simulink model "GS_model"  (R2018b)
settings: Solver=ode5  StartTime=0.0  StopTime=SimuStopTime  FixedStep=T_Simu  RelTol=1e-3
InitFcn:
  | Initial
undefined symbols (not defined in the file or in its folder): Aba10, Aba20, aeroCIP2006_S, aeroCIP2006_X, aeroCIP2006_Y, Agl0, Ass_kS, Ass_n1, Ass_n2, Ass_n3, Ass_n4, Ass_Noise, Ass_R, Ass_Resolution, Ass_TmOrder, AssA_Fix_Abs, AssB_Fix_Abs, AssC_Fix_Abs, AssD_Fix_Abs, AssE_Fix_Aps, AssF_Fix_Aps, C, c_max, c_min, Cd, CenterOfFigNX, CenterOfFigNY, CenterOfFigNZ, CenterOfFigP1, CenterOfFigP2, CenterOfFigPX, CenterOfFigPY, CenterOfFigPZ, Cmu, Crou, DEG2RAD, DiscIntNeverNeededParam, Eg_Dir, Eg_F, Eg_PrepareTime, Eg_r_L_L, Fw_Abf, Fw_Hmax, Fw_J, Fw_Spd0, Fw_Tmax, git_hash_BaseLine, git_hash_Project, Gnss_Noise_Pos, Gnss_Noise_Vel, Gnss_PropgationTime, GyroA_Fix_Abg, GyroA_Noise, GyroB_Fix_Abg, GyroB_Noise, GyroC_Fix_Abg, GyroC_Noise, GyroD_Fix_Abg, GyroD_Noise, h ... (+94)
libraries: simulink x308, sharedutil x46, aerolibutil x37, sharedtransform x31, vrlib x14, aerolibgravity2 x2
(part 6 of 20)

== system GS_model/Subsystem2/Subsystem/Actuator/Engine/Subsystem1/Subsystem ==
  note: Dir_Choice/Switch/X/Y/Z
  Eg_Dir0 : Inport
  Eg_Dir_Set : Inport  Port=2
  Num : Inport  Port=3
  Compare To Constant : simulink/Logic and Bit Operations/Compare To Constant  relop===  const=0  OutDataTypeStr=boolean
  Demux : Demux  Outputs=[1;4]
  Demux5 : Demux  Outputs=[1;3]
  Logical Operator : Logic  Operator=OR  AllPortsSameDT=off  OutDataTypeStr=boolean
  Normalize Vector : vrlib/Utilities/Normalize Vector  maxzero=0
  Relational Operator1 : RelationalOperator  Operator===  OutDataTypeStr=boolean  RndMeth=Simplest
  Switch : Switch  Criteria=u2 > Threshold
  Triggered Subsystem1 : Subsystem  TreatAsAtomicUnit=on
      mask Display: disp('FWChoice')
  Eg_Dir : Outport
  wires:
  Normalize Vector/1 -> Eg_Dir/1
  Relational Operator1/1 -> Logical Operator/1
  Compare To Constant/1 -> Logical Operator/2
  Eg_Dir_Set/1 -> Demux/1
  Demux5/1 -> Switch/2
  Eg_Dir0/1 -> Switch/3
  Demux/2 -> Triggered Subsystem1/1(In1)
  Switch/1 -> Normalize Vector/1
  Logical Operator/1 -> Triggered Subsystem1/Enable
  Triggered Subsystem1/1(Out1) -> Demux5/1
  Num/1 -> Relational Operator1/1
  Demux5/2 -> Switch/1
  Demux/1 -> Compare To Constant/1, Relational Operator1/2

== system GS_model/Subsystem2/Subsystem/Actuator/Engine/Subsystem1/Subsystem1 ==
  note: F_Choice/Switch/Value
  Eg_F0 : Inport
  Eg_F_Set : Inport  Port=2
  Num : Inport  Port=3
  Compare To Constant : simulink/Logic and Bit Operations/Compare To Constant  relop===  const=0  OutDataTypeStr=boolean
  Demux : Demux  Outputs=[1;2]
  Demux5 : Demux  Outputs=[1;1]
  Logical Operator : Logic  Operator=OR  AllPortsSameDT=off  OutDataTypeStr=boolean
  Relational Operator1 : RelationalOperator  Operator===  OutDataTypeStr=boolean  RndMeth=Simplest
  Switch : Switch  Criteria=u2 > Threshold
  Triggered Subsystem1 : Subsystem  TreatAsAtomicUnit=on
      mask Display: disp('FWChoice')
  Eg_F : Outport
  wires:
  Demux/1 -> Relational Operator1/2, Compare To Constant/1
  Demux5/2 -> Switch/1
  Num/1 -> Relational Operator1/1
  Triggered Subsystem1/1(Out1) -> Demux5/1
  Logical Operator/1 -> Triggered Subsystem1/Enable
  Switch/1 -> Eg_F/1
  Demux/2 -> Triggered Subsystem1/1(In1)
  Eg_F0/1 -> Switch/3
  Demux5/1 -> Switch/2
  Eg_F_Set/1 -> Demux/1
  Compare To Constant/1 -> Logical Operator/2
  Relational Operator1/1 -> Logical Operator/1

== system GS_model/Subsystem2/Subsystem/Actuator/Engine/Subsystem1/Subsystem2 ==
  note: FirePause_Choice/Switch/Value
  Eg_F_Set : Inport
  Num : Inport  Port=2
  Compare To Constant : simulink/Logic and Bit Operations/Compare To Constant  relop===  const=0  OutDataTypeStr=boolean
  Demux : Demux  Outputs=[1;2]
  Logical Operator : Logic  Operator=OR  AllPortsSameDT=off  OutDataTypeStr=boolean
  Relational Operator1 : RelationalOperator  Operator===  OutDataTypeStr=boolean  RndMeth=Simplest
  Triggered Subsystem1 : Subsystem  TreatAsAtomicUnit=on
      mask Display: disp('FWChoice')
  Eg_FirePause : Outport
  wires:
  Relational Operator1/1 -> Logical Operator/1
  Compare To Constant/1 -> Logical Operator/2
  Eg_F_Set/1 -> Demux/1
  Demux/2 -> Triggered Subsystem1/1(In1)
  Logical Operator/1 -> Triggered Subsystem1/Enable
  Triggered Subsystem1/1(Out1) -> Eg_FirePause/1
  Num/1 -> Relational Operator1/1
  Demux/1 -> Compare To Constant/1, Relational Operator1/2

== system GS_model/Subsystem2/Subsystem/Actuator/FlyWheel/FwAModel1/FWDataSourceChoice ==
  note: 1 -- FW_Spd_422
      | 2 -- FW_Spd_UDP
      | 3 -- FW_Spd_FC
      |
      | 4 -- FW_T_422
      | 5 -- FW_T_UDP
      | 6 -- FW_T_FC
      |
      | 7 -- FW_Mode_422
      | 8 -- FW_Mode_UDP
      | 9 -- FW_Mode_FC
  FW_Cmd : Inport
  TC_FW_DelaySet : Inport  Port=2
  DelayModel : Subsystem
  Demux : Demux  Outputs=3
  Mux1 : Mux  Inputs=3
  Cmd_Mode/Spd/T : Outport
  Cmd_Mode : Outport  Port=2
  wires:
  Mux1/1 -> Cmd_Mode/Spd/T/1
  DelayModel/3(Cmd_T) -> Mux1/3
  DelayModel/1(Cmd_Mode) -> Mux1/1, Cmd_Mode/1
  DelayModel/2(Cmd_Spd) -> Mux1/2
  TC_FW_DelaySet/1 -> DelayModel/1(TC_FW_Delay)
  FW_Cmd/1 -> Demux/1
  Demux/3 -> DelayModel/4(FW_Cmd_T)
  Demux/2 -> DelayModel/3(FW_Cmd_Spd)
  Demux/1 -> DelayModel/2(FW_Cmd_Mode)

== system GS_model/Subsystem2/Subsystem/Actuator/FlyWheel/FwAModel1/FWMath&ErrModel ==
  Cmd_Mode : Inport
  TC_FW_TSet : Inport  Port=2
  TC_FW_SpdSet : Inport  Port=3
  TC_FW_ModeSet : Inport  Port=4
  TC_FWErr_Spd_Op : Inport  Port=5
  TC_FWErr_T_Op : Inport  Port=6
  FwSpd : Inport  Port=7
  FwT : Inport  Port=8
  FWNum : Inport  Port=9
  Mux : Mux  Inputs=3
  Subsystem1 : Subsystem
      mask Display: disp('FWTErrModel')
  Subsystem2 : Subsystem
      mask Display: disp('FWSpdErrModel')
  Subsystem4 : Subsystem
      mask Display: disp('FWModeErrModel')
  TM_FW : Outport
  Dyn_FW_T : Outport  Port=2
  Dyn_FW_Spd : Outport  Port=3
  wires:
  FwSpd/1 -> Subsystem2/1(Fb_FW_Spd), Dyn_FW_Spd/1
  TC_FW_TSet/1 -> Subsystem1/2(TC_FW_TSet)
  TC_FW_SpdSet/1 -> Subsystem2/2(TC_FW_SpdSet)
  TC_FW_ModeSet/1 -> Subsystem4/3(TC_FW_ModeSet)
  FwT/1 -> Subsystem1/1(Fb_FW_T), Dyn_FW_T/1
  Cmd_Mode/1 -> Subsystem4/2(FW_Mode)
  TC_FWErr_Spd_Op/1 -> Subsystem2/4(TC_FWErr_SpdOp)
  TC_FWErr_T_Op/1 -> Subsystem1/4(TC_FWErr_TOp)
  Mux/1 -> TM_FW/1
  Subsystem2/1(TM_FW_Spd) -> Mux/2
  Subsystem4/1(Fb_FW_Mode) -> Mux/1
  Subsystem1/1(TM_FW_T) -> Mux/3
  FWNum/1 -> Subsystem1/3(FWNum), Subsystem2/3(FWNum), Subsystem4/1(FWNum)

== system GS_model/Subsystem2/Subsystem/Actuator/FlyWheel/FwAModel2/FWDataSourceChoice ==
  note: 1 -- FW_Spd_422
      | 2 -- FW_Spd_UDP
      | 3 -- FW_Spd_FC
      |
      | 4 -- FW_T_422
      | 5 -- FW_T_UDP
      | 6 -- FW_T_FC
      |
      | 7 -- FW_Mode_422
      | 8 -- FW_Mode_UDP
      | 9 -- FW_Mode_FC
  FW_Cmd : Inport
  TC_FW_DelaySet : Inport  Port=2
  DelayModel : Subsystem
  Demux : Demux  Outputs=3
  Mux1 : Mux  Inputs=3
  Cmd_Mode/Spd/T : Outport
  Cmd_Mode : Outport  Port=2
  wires:
  Demux/1 -> DelayModel/2(FW_Cmd_Mode)
  Demux/2 -> DelayModel/3(FW_Cmd_Spd)
  Demux/3 -> DelayModel/4(FW_Cmd_T)
  FW_Cmd/1 -> Demux/1
  TC_FW_DelaySet/1 -> DelayModel/1(TC_FW_Delay)
  DelayModel/2(Cmd_Spd) -> Mux1/2
  DelayModel/1(Cmd_Mode) -> Cmd_Mode/1, Mux1/1
  DelayModel/3(Cmd_T) -> Mux1/3
  Mux1/1 -> Cmd_Mode/Spd/T/1

== system GS_model/Subsystem2/Subsystem/Actuator/FlyWheel/FwAModel2/FWMath&ErrModel ==
  Cmd_Mode : Inport
  TC_FW_TSet : Inport  Port=2
  TC_FW_SpdSet : Inport  Port=3
  TC_FW_ModeSet : Inport  Port=4
  TC_FWErr_Spd_Op : Inport  Port=5
  TC_FWErr_T_Op : Inport  Port=6
  FwSpd : Inport  Port=7
  FwT : Inport  Port=8
  FWNum : Inport  Port=9
  Mux : Mux  Inputs=3
  Subsystem1 : Subsystem
      mask Display: disp('FWTErrModel')
  Subsystem2 : Subsystem
      mask Display: disp('FWSpdErrModel')
  Subsystem4 : Subsystem
      mask Display: disp('FWModeErrModel')
  TM_FW : Outport
  Dyn_FW_T : Outport  Port=2
  Dyn_FW_Spd : Outport  Port=3
  wires:
  FWNum/1 -> Subsystem4/1(FWNum), Subsystem2/3(FWNum), Subsystem1/3(FWNum)
  Subsystem1/1(TM_FW_T) -> Mux/3
  Subsystem4/1(Fb_FW_Mode) -> Mux/1
  Subsystem2/1(TM_FW_Spd) -> Mux/2
  Mux/1 -> TM_FW/1
  TC_FWErr_T_Op/1 -> Subsystem1/4(TC_FWErr_TOp)
  TC_FWErr_Spd_Op/1 -> Subsystem2/4(TC_FWErr_SpdOp)
  Cmd_Mode/1 -> Subsystem4/2(FW_Mode)
  FwT/1 -> Dyn_FW_T/1, Subsystem1/1(Fb_FW_T)
  TC_FW_ModeSet/1 -> Subsystem4/3(TC_FW_ModeSet)
  TC_FW_SpdSet/1 -> Subsystem2/2(TC_FW_SpdSet)
  TC_FW_TSet/1 -> Subsystem1/2(TC_FW_TSet)
  FwSpd/1 -> Dyn_FW_Spd/1, Subsystem2/1(Fb_FW_Spd)

== system GS_model/Subsystem2/Subsystem/Actuator/FlyWheel/FwAModel3/FWDataSourceChoice ==
  note: 1 -- FW_Spd_422
      | 2 -- FW_Spd_UDP
      | 3 -- FW_Spd_FC
      |
      | 4 -- FW_T_422
      | 5 -- FW_T_UDP
      | 6 -- FW_T_FC
      |
      | 7 -- FW_Mode_422
      | 8 -- FW_Mode_UDP
      | 9 -- FW_Mode_FC
  FW_Cmd : Inport
  TC_FW_DelaySet : Inport  Port=2
  DelayModel : Subsystem
  Demux : Demux  Outputs=3
  Mux1 : Mux  Inputs=3
  Cmd_Mode/Spd/T : Outport
  Cmd_Mode : Outport  Port=2
  wires:
  Mux1/1 -> Cmd_Mode/Spd/T/1
  DelayModel/3(Cmd_T) -> Mux1/3
  DelayModel/1(Cmd_Mode) -> Mux1/1, Cmd_Mode/1
  DelayModel/2(Cmd_Spd) -> Mux1/2
  TC_FW_DelaySet/1 -> DelayModel/1(TC_FW_Delay)
  FW_Cmd/1 -> Demux/1
  Demux/3 -> DelayModel/4(FW_Cmd_T)
  Demux/2 -> DelayModel/3(FW_Cmd_Spd)
  Demux/1 -> DelayModel/2(FW_Cmd_Mode)

== system GS_model/Subsystem2/Subsystem/Actuator/FlyWheel/FwAModel3/FWMath&ErrModel ==
  Cmd_Mode : Inport
  TC_FW_TSet : Inport  Port=2
  TC_FW_SpdSet : Inport  Port=3
  TC_FW_ModeSet : Inport  Port=4
  TC_FWErr_Spd_Op : Inport  Port=5
  TC_FWErr_T_Op : Inport  Port=6
  FwSpd : Inport  Port=7
  FwT : Inport  Port=8
  FWNum : Inport  Port=9
  Mux : Mux  Inputs=3
  Subsystem1 : Subsystem
      mask Display: disp('FWTErrModel')
  Subsystem2 : Subsystem
      mask Display: disp('FWSpdErrModel')
  Subsystem4 : Subsystem
      mask Display: disp('FWModeErrModel')
  TM_FW : Outport
  Dyn_FW_T : Outport  Port=2
  Dyn_FW_Spd : Outport  Port=3
  wires:
  FwSpd/1 -> Subsystem2/1(Fb_FW_Spd), Dyn_FW_Spd/1
  TC_FW_TSet/1 -> Subsystem1/2(TC_FW_TSet)
  TC_FW_SpdSet/1 -> Subsystem2/2(TC_FW_SpdSet)
  TC_FW_ModeSet/1 -> Subsystem4/3(TC_FW_ModeSet)
  FwT/1 -> Subsystem1/1(Fb_FW_T), Dyn_FW_T/1
  Cmd_Mode/1 -> Subsystem4/2(FW_Mode)
  TC_FWErr_Spd_Op/1 -> Subsystem2/4(TC_FWErr_SpdOp)
  TC_FWErr_T_Op/1 -> Subsystem1/4(TC_FWErr_TOp)
  Mux/1 -> TM_FW/1
  Subsystem2/1(TM_FW_Spd) -> Mux/2
  Subsystem4/1(Fb_FW_Mode) -> Mux/1
  Subsystem1/1(TM_FW_T) -> Mux/3
  FWNum/1 -> Subsystem1/3(FWNum), Subsystem2/3(FWNum), Subsystem4/1(FWNum)

== system GS_model/Subsystem2/Subsystem/Actuator/FlyWheel/FwAModel4/FWDataSourceChoice ==
  note: 1 -- FW_Spd_422
      | 2 -- FW_Spd_UDP
      | 3 -- FW_Spd_FC
      |
      | 4 -- FW_T_422
      | 5 -- FW_T_UDP
      | 6 -- FW_T_FC
      |
      | 7 -- FW_Mode_422
      | 8 -- FW_Mode_UDP
      | 9 -- FW_Mode_FC
  FW_Cmd : Inport
  TC_FW_DelaySet : Inport  Port=2
  DelayModel : Subsystem
  Demux : Demux  Outputs=3
  Mux1 : Mux  Inputs=3
  Cmd_Mode/Spd/T : Outport
  Cmd_Mode : Outport  Port=2
  wires:
  Demux/1 -> DelayModel/2(FW_Cmd_Mode)
  Demux/2 -> DelayModel/3(FW_Cmd_Spd)
  Demux/3 -> DelayModel/4(FW_Cmd_T)
  FW_Cmd/1 -> Demux/1
  TC_FW_DelaySet/1 -> DelayModel/1(TC_FW_Delay)
  DelayModel/2(Cmd_Spd) -> Mux1/2
  DelayModel/1(Cmd_Mode) -> Cmd_Mode/1, Mux1/1
  DelayModel/3(Cmd_T) -> Mux1/3
  Mux1/1 -> Cmd_Mode/Spd/T/1

== system GS_model/Subsystem2/Subsystem/Actuator/FlyWheel/FwAModel4/FWMath&ErrModel ==
  Cmd_Mode : Inport
  TC_FW_TSet : Inport  Port=2
  TC_FW_SpdSet : Inport  Port=3
  TC_FW_ModeSet : Inport  Port=4
  TC_FWErr_Spd_Op : Inport  Port=5
  TC_FWErr_T_Op : Inport  Port=6
  FwSpd : Inport  Port=7
  FwT : Inport  Port=8
  FWNum : Inport  Port=9
  Mux : Mux  Inputs=3
  Subsystem1 : Subsystem
      mask Display: disp('FWTErrModel')
  Subsystem2 : Subsystem
      mask Display: disp('FWSpdErrModel')
  Subsystem4 : Subsystem
      mask Display: disp('FWModeErrModel')
  TM_FW : Outport
  Dyn_FW_T : Outport  Port=2
  Dyn_FW_Spd : Outport  Port=3
  wires:
  FWNum/1 -> Subsystem4/1(FWNum), Subsystem2/3(FWNum), Subsystem1/3(FWNum)
  Subsystem1/1(TM_FW_T) -> Mux/3
  Subsystem4/1(Fb_FW_Mode) -> Mux/1
  Subsystem2/1(TM_FW_Spd) -> Mux/2
  Mux/1 -> TM_FW/1
  TC_FWErr_T_Op/1 -> Subsystem1/4(TC_FWErr_TOp)
  TC_FWErr_Spd_Op/1 -> Subsystem2/4(TC_FWErr_SpdOp)
  Cmd_Mode/1 -> Subsystem4/2(FW_Mode)
  FwT/1 -> Dyn_FW_T/1, Subsystem1/1(Fb_FW_T)
  TC_FW_ModeSet/1 -> Subsystem4/3(TC_FW_ModeSet)
  TC_FW_SpdSet/1 -> Subsystem2/2(TC_FW_SpdSet)
  TC_FW_TSet/1 -> Subsystem1/2(TC_FW_TSet)
  FwSpd/1 -> Dyn_FW_Spd/1, Subsystem2/1(Fb_FW_Spd)

== system GS_model/Subsystem2/Subsystem/Actuator/FlyWheel/FwAModel5/FWDataSourceChoice ==
  note: 1 -- FW_Spd_422
      | 2 -- FW_Spd_UDP
      | 3 -- FW_Spd_FC
      |
      | 4 -- FW_T_422
      | 5 -- FW_T_UDP
      | 6 -- FW_T_FC
      |
      | 7 -- FW_Mode_422
      | 8 -- FW_Mode_UDP
      | 9 -- FW_Mode_FC
  FW_Cmd : Inport
  TC_FW_DelaySet : Inport  Port=2
  DelayModel : Subsystem
  Demux : Demux  Outputs=3
  Mux1 : Mux  Inputs=3
  Cmd_Mode/Spd/T : Outport
  Cmd_Mode : Outport  Port=2
  wires:
  Mux1/1 -> Cmd_Mode/Spd/T/1
  DelayModel/3(Cmd_T) -> Mux1/3
  DelayModel/1(Cmd_Mode) -> Mux1/1, Cmd_Mode/1
  DelayModel/2(Cmd_Spd) -> Mux1/2
  TC_FW_DelaySet/1 -> DelayModel/1(TC_FW_Delay)
  FW_Cmd/1 -> Demux/1
  Demux/3 -> DelayModel/4(FW_Cmd_T)
  Demux/2 -> DelayModel/3(FW_Cmd_Spd)
  Demux/1 -> DelayModel/2(FW_Cmd_Mode)

== system GS_model/Subsystem2/Subsystem/Actuator/FlyWheel/FwAModel5/FWMath&ErrModel ==
  Cmd_Mode : Inport
  TC_FW_TSet : Inport  Port=2
  TC_FW_SpdSet : Inport  Port=3
  TC_FW_ModeSet : Inport  Port=4
  TC_FWErr_Spd_Op : Inport  Port=5
  TC_FWErr_T_Op : Inport  Port=6
  FwSpd : Inport  Port=7
  FwT : Inport  Port=8
  FWNum : Inport  Port=9
  Mux : Mux  Inputs=3
  Subsystem1 : Subsystem
      mask Display: disp('FWTErrModel')
  Subsystem2 : Subsystem
      mask Display: disp('FWSpdErrModel')
  Subsystem4 : Subsystem
      mask Display: disp('FWModeErrModel')
  TM_FW : Outport
  Dyn_FW_T : Outport  Port=2
  Dyn_FW_Spd : Outport  Port=3
  wires:
  FwSpd/1 -> Subsystem2/1(Fb_FW_Spd), Dyn_FW_Spd/1
  TC_FW_TSet/1 -> Subsystem1/2(TC_FW_TSet)
  TC_FW_SpdSet/1 -> Subsystem2/2(TC_FW_SpdSet)
  TC_FW_ModeSet/1 -> Subsystem4/3(TC_FW_ModeSet)
  FwT/1 -> Subsystem1/1(Fb_FW_T), Dyn_FW_T/1
  Cmd_Mode/1 -> Subsystem4/2(FW_Mode)
  TC_FWErr_Spd_Op/1 -> Subsystem2/4(TC_FWErr_SpdOp)
  TC_FWErr_T_Op/1 -> Subsystem1/4(TC_FWErr_TOp)
  Mux/1 -> TM_FW/1
  Subsystem2/1(TM_FW_Spd) -> Mux/2
  Subsystem4/1(Fb_FW_Mode) -> Mux/1
  Subsystem1/1(TM_FW_T) -> Mux/3
  FWNum/1 -> Subsystem1/3(FWNum), Subsystem2/3(FWNum), Subsystem4/1(FWNum)

== system GS_model/Subsystem2/Subsystem/Actuator/FlyWheel/FwAModel6/FWDataSourceChoice ==
  note: 1 -- FW_Spd_422
      | 2 -- FW_Spd_UDP
      | 3 -- FW_Spd_FC
      |
      | 4 -- FW_T_422
      | 5 -- FW_T_UDP
      | 6 -- FW_T_FC
      |
      | 7 -- FW_Mode_422
      | 8 -- FW_Mode_UDP
      | 9 -- FW_Mode_FC
  FW_Cmd : Inport
  TC_FW_DelaySet : Inport  Port=2
  DelayModel : Subsystem
  Demux : Demux  Outputs=3
  Mux1 : Mux  Inputs=3
  Cmd_Mode/Spd/T : Outport
  Cmd_Mode : Outport  Port=2
  wires:
  Demux/1 -> DelayModel/2(FW_Cmd_Mode)
  Demux/2 -> DelayModel/3(FW_Cmd_Spd)
  Demux/3 -> DelayModel/4(FW_Cmd_T)
  FW_Cmd/1 -> Demux/1
  TC_FW_DelaySet/1 -> DelayModel/1(TC_FW_Delay)
  DelayModel/2(Cmd_Spd) -> Mux1/2
  DelayModel/1(Cmd_Mode) -> Cmd_Mode/1, Mux1/1
  DelayModel/3(Cmd_T) -> Mux1/3
  Mux1/1 -> Cmd_Mode/Spd/T/1

== system GS_model/Subsystem2/Subsystem/Actuator/FlyWheel/FwAModel6/FWMath&ErrModel ==
  Cmd_Mode : Inport
  TC_FW_TSet : Inport  Port=2
  TC_FW_SpdSet : Inport  Port=3
  TC_FW_ModeSet : Inport  Port=4
  TC_FWErr_Spd_Op : Inport  Port=5
  TC_FWErr_T_Op : Inport  Port=6
  FwSpd : Inport  Port=7
  FwT : Inport  Port=8
  FWNum : Inport  Port=9
  Mux : Mux  Inputs=3
  Subsystem1 : Subsystem
      mask Display: disp('FWTErrModel')
  Subsystem2 : Subsystem
      mask Display: disp('FWSpdErrModel')
  Subsystem4 : Subsystem
      mask Display: disp('FWModeErrModel')
  TM_FW : Outport
  Dyn_FW_T : Outport  Port=2
  Dyn_FW_Spd : Outport  Port=3
  wires:
  FWNum/1 -> Subsystem4/1(FWNum), Subsystem2/3(FWNum), Subsystem1/3(FWNum)
  Subsystem1/1(TM_FW_T) -> Mux/3
  Subsystem4/1(Fb_FW_Mode) -> Mux/1
  Subsystem2/1(TM_FW_Spd) -> Mux/2
  Mux/1 -> TM_FW/1
  TC_FWErr_T_Op/1 -> Subsystem1/4(TC_FWErr_TOp)
  TC_FWErr_Spd_Op/1 -> Subsystem2/4(TC_FWErr_SpdOp)
  Cmd_Mode/1 -> Subsystem4/2(FW_Mode)
  FwT/1 -> Dyn_FW_T/1, Subsystem1/1(Fb_FW_T)
  TC_FW_ModeSet/1 -> Subsystem4/3(TC_FW_ModeSet)
  TC_FW_SpdSet/1 -> Subsystem2/2(TC_FW_SpdSet)
  TC_FW_TSet/1 -> Subsystem1/2(TC_FW_TSet)
  FwSpd/1 -> Dyn_FW_Spd/1, Subsystem2/1(Fb_FW_Spd)

== system GS_model/Subsystem2/Subsystem/Actuator/FlyWheel/FwAModel7/FwMathModel ==
  note: 1--转矩模式
      | 2--转速模式
  Cmd_Mode : Inport
  Cmd_Spd : Inport  Port=2
  Cmd_T : Inport  Port=3
  Reset : Inport  Port=4
  FwH0 : Inport  Port=5
  Tc_Fw_FricCoff : Inport  Port=6
  10mN--6000rpm : Gain  Gain=0.01./Fw_Hmax
  Compare To Constant : simulink/Logic and Bit Operations/Compare To Constant  relop===  const=2.0  OutDataTypeStr=boolean
  Compare To Constant1 : simulink/Logic and Bit Operations/Compare To Constant  relop===  const=1.0  OutDataTypeStr=boolean
  Data Type Conversion : DataTypeConversion  OutDataTypeStr=double
  Data Type Conversion1 : DataTypeConversion  OutDataTypeStr=double
  Gain2 : Gain  Gain=1./Fw_J
  Gain3 : Gain  Gain=1./Fw_J
  Integrator Limited1 : Integrator  ExternalReset=level  InitialConditionSource=external  LimitOutput=on  UpperSaturationLimit=Fw_Hmax  LowerSaturationLimit=-Fw_Hmax
  K : Gain  Gain=Fw_J  SaturateOnIntegerOverflow=on  OutDataTypeStr=Inherit: Same as input  ParamDataTypeStr=Inherit: Same as input
  Memory : Memory  InheritSampleTime=on
  Product : Product
  Product1 : Product
  Product2 : Product
  RPM2RadPerSec : Gain  Gain=RPM2RadPerSec  SaturateOnIntegerOverflow=on  OutDataTypeStr=Inherit: Same as input  ParamDataTypeStr=Inherit: Same as input
  RadPerSec2RPM : Gain  Gain=RadPerSec2RPM  SaturateOnIntegerOverflow=on  OutDataTypeStr=Inherit: Same as input  ParamDataTypeStr=Inherit: Same as input
  Sum : Sum  Inputs=|+-  SaturateOnIntegerOverflow=on
  Sum1 : Sum  Inputs=++|
  Sum2 : Sum  Inputs=|+-  SaturateOnIntegerOverflow=on
  Sum3 : Sum  Inputs=|+-
  T=0.1 : Gain  Gain=1/0.1  SaturateOnIntegerOverflow=on  OutDataTypeStr=Inherit: Same as input  ParamDataTypeStr=Inherit: Same as input
  T_lim1 : Saturate  UpperLimit=Fw_Tmax  LowerLimit=-Fw_Tmax  LinearizeAsGain=off
  T_lim2 : Saturate  UpperLimit=Fw_Tmax  LowerLimit=-Fw_Tmax  LinearizeAsGain=off
  T_lim3 : Saturate  UpperLimit=Fw_Tmax  LowerLimit=-Fw_Tmax  LinearizeAsGain=off
  dw : Gain  Gain=1/T_Simu  SaturateOnIntegerOverflow=on  OutDataTypeStr=Inherit: Same as input  ParamDataTypeStr=Inherit: Same as input
  Fw_Spd_out : Outport
  Fw_T_out : Outport  Port=2
  wires:
  Gain3/1 -> Sum/2
  Gain2/1 -> RadPerSec2RPM/1
  dw/1 -> T_lim1/1
  K/1 -> T_lim3/1
  Memory/1 -> Sum2/2
  FwH0/1 -> Integrator Limited1/3
  Product2/1 -> Sum3/2
  Cmd_Mode/1 -> Compare To Constant1/1, Compare To Constant/1
  Sum2/1 -> dw/1
  T=0.1/1 -> K/1
  Reset/1 -> Integrator Limited1/2
  Product1/1 -> Sum1/1
  10mN--6000rpm/1 -> Product2/2
  Integrator Limited1/1 -> Sum2/1, Gain2/1, 10mN--6000rpm/1, Gain3/1, Memory/1
  Compare To Constant/1 -> Data Type Conversion/1
  Sum/1 -> T=0.1/1
  Data Type Conversion1/1 -> Product1/2
  Tc_Fw_FricCoff/1 -> Product2/1
  Cmd_T/1 -> T_lim2/1
  Sum3/1 -> Integrator Limited1/1
  Cmd_Spd/1 -> RPM2RadPerSec/1
  T_lim2/1 -> Product1/1
  Product/1 -> Sum1/2
  Sum1/1 -> Sum3/1
  Data Type Conversion/1 -> Product/1
  Compare To Constant1/1 -> Data Type Conversion1/1
  RPM2RadPerSec/1 -> Sum/1
  RadPerSec2RPM/1 -> Fw_Spd_out/1
  T_lim1/1 -> Fw_T_out/1
  T_lim3/1 -> Product/2

== system GS_model/Subsystem2/Subsystem/Actuator/Magnetorquer/Mt_MathModel/MtA1 ==
  Tc_Mt : Inport
  Cmd : Inport  Port=2
  Mt_Num : Inport  Port=3
  >=<0 to 012 : Subsystem
  Abs3 : Abs
  Compare To Constant : simulink/Logic and Bit Operations/Compare To Constant  relop===  const=0  OutDataTypeStr=boolean
  Constant : Constant  Value=Mt_Cur2M
  Constant1 : Constant  Value=Mt_M2Cur
  Constant2 : Constant  Value=Mt_max_M
  Demux : Demux  Outputs=2
  Demux3 : Demux  Outputs=[1;2]
  Demux8 : Demux  Outputs=2
  If Action Subsystem3 : Subsystem  TreatAsAtomicUnit=on
  If Action Subsystem4 : Subsystem  TreatAsAtomicUnit=on
  If1 : If  IfExpression=u1 == 1
  Index Vector : MultiPortSwitch  Inputs=1
  Index Vector1 : MultiPortSwitch  Inputs=1
  Logical Operator : Logic  Operator=OR  AllPortsSameDT=off  OutDataTypeStr=boolean
  Mag_CmdCal : Subsystem
  Merge1 : Merge
  Mux : Mux  Inputs=2
  Mux1 : Mux  Inputs=2
  Product2 : Product
  Product3 : Product
  Relational Operator5 : RelationalOperator  Operator===  OutDataTypeStr=boolean  RndMeth=Simplest
  Saturation : MATLAB Function  TreatAsAtomicUnit=on
  Triggered Subsystem6 : Subsystem  TreatAsAtomicUnit=on
  Mc_Mt : Outport
  Tm_Mt : Outport  Port=2
  Cmd_Mt : Outport  Port=3
  wires:
  Product3/1 -> Mux1/1
  Index Vector/1 -> Product3/1
  Abs3/1 -> Product3/2
  Mag_CmdCal/1("Cmd_Curr ") -> If Action Subsystem3/1(In1)
  >=<0 to 012/1(Out1) -> Mux1/2
  If Action Subsystem4/1(Out1) -> Merge1/1
  Tc_Mt/1 -> Demux3/1
  Demux8/1 -> If1/1
  If Action Subsystem3/1(Out1) -> Merge1/2
  Demux3/1 -> Compare To Constant/1, Relational Operator5/2
  Demux3/2 -> Triggered Subsystem6/1(In1)
  Triggered Subsystem6/1(Out1) -> Demux8/1
  If1/2 -> If Action Subsystem3/Action
  If1/1 -> If Action Subsystem4/Action
  Mag_CmdCal/2(Cmd_Dirr) -> Mux/2
  Mux/1 -> Cmd_Mt/1
  Mux1/1 -> Tm_Mt/1
  Demux8/2 -> If Action Subsystem4/1(In1)
  Constant1/1 -> Index Vector/2
  Mt_Num/1 -> Index Vector/1, Index Vector1/1, Saturation/2(Num), Relational Operator5/1
  Relational Operator5/1 -> Logical Operator/2
  Logical Operator/1 -> Triggered Subsystem6/Enable
  Compare To Constant/1 -> Logical Operator/1
  Index Vector1/1 -> Product2/1
  Merge1/1 -> Product2/2
  Constant/1 -> Index Vector1/2
  Product2/1 -> Saturation/1(Mc_In)
  Demux/1 -> Mag_CmdCal/1(Cmd_Dir)
  Demux/2 -> Mux/1, Mag_CmdCal/2(Cmd_Cur)
  Cmd/1 -> Demux/1
  Saturation/1(Mc_Out) -> Mc_Mt/1, >=<0 to 012/1(In1), Abs3/1
  Constant2/1 -> Saturation/3(Mt_max_M)

== system GS_model/Subsystem2/Subsystem/Actuator/Magnetorquer/Mt_MathModel/MtA2 ==
  Tc_Mt : Inport
  Cmd : Inport  Port=2
  Mt_Num : Inport  Port=3
  >=<0 to 012 : Subsystem
  Abs3 : Abs
  Compare To Constant : simulink/Logic and Bit Operations/Compare To Constant  relop===  const=0  OutDataTypeStr=boolean
  Constant : Constant  Value=Mt_Cur2M
  Constant1 : Constant  Value=Mt_M2Cur
  Constant2 : Constant  Value=Mt_max_M
  Demux : Demux  Outputs=2
  Demux3 : Demux  Outputs=[1;2]
  Demux8 : Demux  Outputs=2
  If Action Subsystem3 : Subsystem  TreatAsAtomicUnit=on
  If Action Subsystem4 : Subsystem  TreatAsAtomicUnit=on
  If1 : If  IfExpression=u1 == 1
  Index Vector : MultiPortSwitch  Inputs=1
  Index Vector1 : MultiPortSwitch  Inputs=1
  Logical Operator : Logic  Operator=OR  AllPortsSameDT=off  OutDataTypeStr=boolean
  Mag_CmdCal : Subsystem
  Merge1 : Merge
  Mux : Mux  Inputs=2
  Mux1 : Mux  Inputs=2
  Product2 : Product
  Product3 : Product
  Relational Operator5 : RelationalOperator  Operator===  OutDataTypeStr=boolean  RndMeth=Simplest
  Saturation : MATLAB Function  TreatAsAtomicUnit=on
  Triggered Subsystem6 : Subsystem  TreatAsAtomicUnit=on
  Mc_Mt : Outport
  Tm_Mt : Outport  Port=2
  Cmd_Mt : Outport  Port=3
  wires:
  Constant2/1 -> Saturation/3(Mt_max_M)
  Saturation/1(Mc_Out) -> Abs3/1, >=<0 to 012/1(In1), Mc_Mt/1
  Cmd/1 -> Demux/1
  Demux/2 -> Mag_CmdCal/2(Cmd_Cur), Mux/1
  Demux/1 -> Mag_CmdCal/1(Cmd_Dir)
  Product2/1 -> Saturation/1(Mc_In)
  Constant/1 -> Index Vector1/2
  Merge1/1 -> Product2/2
  Index Vector1/1 -> Product2/1
  Compare To Constant/1 -> Logical Operator/1
  Logical Operator/1 -> Triggered Subsystem6/Enable
  Relational Operator5/1 -> Logical Operator/2
  Mt_Num/1 -> Relational Operator5/1, Saturation/2(Num), Index Vector1/1, Index Vector/1
  Constant1/1 -> Index Vector/2
  Demux8/2 -> If Action Subsystem4/1(In1)
  Mux1/1 -> Tm_Mt/1
  Mux/1 -> Cmd_Mt/1
  Mag_CmdCal/2(Cmd_Dirr) -> Mux/2
  If1/1 -> If Action Subsystem4/Action
  If1/2 -> If Action Subsystem3/Action
  Triggered Subsystem6/1(Out1) -> Demux8/1
  Demux3/2 -> Triggered Subsystem6/1(In1)
  Demux3/1 -> Relational Operator5/2, Compare To Constant/1
  If Action Subsystem3/1(Out1) -> Merge1/2
  Demux8/1 -> If1/1
  Tc_Mt/1 -> Demux3/1
  If Action Subsystem4/1(Out1) -> Merge1/1
  >=<0 to 012/1(Out1) -> Mux1/2
  Mag_CmdCal/1("Cmd_Curr ") -> If Action Subsystem3/1(In1)
  Abs3/1 -> Product3/2
  Index Vector/1 -> Product3/1
  Product3/1 -> Mux1/1

== system GS_model/Subsystem2/Subsystem/Actuator/Magnetorquer/Mt_MathModel/MtA3 ==
  Tc_Mt : Inport
  Cmd : Inport  Port=2
  Mt_Num : Inport  Port=3
  >=<0 to 012 : Subsystem
  Abs3 : Abs
  Compare To Constant : simulink/Logic and Bit Operations/Compare To Constant  relop===  const=0  OutDataTypeStr=boolean
  Constant : Constant  Value=Mt_Cur2M
  Constant1 : Constant  Value=Mt_M2Cur
  Constant2 : Constant  Value=Mt_max_M
  Demux : Demux  Outputs=2
  Demux3 : Demux  Outputs=[1;2]
  Demux8 : Demux  Outputs=2
  If Action Subsystem3 : Subsystem  TreatAsAtomicUnit=on
  If Action Subsystem4 : Subsystem  TreatAsAtomicUnit=on
  If1 : If  IfExpression=u1 == 1
  Index Vector : MultiPortSwitch  Inputs=1
  Index Vector1 : MultiPortSwitch  Inputs=1
  Logical Operator : Logic  Operator=OR  AllPortsSameDT=off  OutDataTypeStr=boolean
  Mag_CmdCal : Subsystem
  Merge1 : Merge
  Mux : Mux  Inputs=2
  Mux1 : Mux  Inputs=2
  Product2 : Product
  Product3 : Product
  Relational Operator5 : RelationalOperator  Operator===  OutDataTypeStr=boolean  RndMeth=Simplest
  Saturation : MATLAB Function  TreatAsAtomicUnit=on
  Triggered Subsystem6 : Subsystem  TreatAsAtomicUnit=on
  Mc_Mt : Outport
  Tm_Mt : Outport  Port=2
  Cmd_Mt : Outport  Port=3
  wires:
  Product3/1 -> Mux1/1
  Index Vector/1 -> Product3/1
  Abs3/1 -> Product3/2
  Mag_CmdCal/1("Cmd_Curr ") -> If Action Subsystem3/1(In1)
  >=<0 to 012/1(Out1) -> Mux1/2
  If Action Subsystem4/1(Out1) -> Merge1/1
  Tc_Mt/1 -> Demux3/1
  Demux8/1 -> If1/1
  If Action Subsystem3/1(Out1) -> Merge1/2
  Demux3/1 -> Compare To Constant/1, Relational Operator5/2
  Demux3/2 -> Triggered Subsystem6/1(In1)
  Triggered Subsystem6/1(Out1) -> Demux8/1
  If1/2 -> If Action Subsystem3/Action
  If1/1 -> If Action Subsystem4/Action
  Mag_CmdCal/2(Cmd_Dirr) -> Mux/2
  Mux/1 -> Cmd_Mt/1
  Mux1/1 -> Tm_Mt/1
  Demux8/2 -> If Action Subsystem4/1(In1)
  Constant1/1 -> Index Vector/2
  Mt_Num/1 -> Index Vector/1, Index Vector1/1, Saturation/2(Num), Relational Operator5/1
  Relational Operator5/1 -> Logical Operator/2
  Logical Operator/1 -> Triggered Subsystem6/Enable
  Compare To Constant/1 -> Logical Operator/1
  Index Vector1/1 -> Product2/1
  Merge1/1 -> Product2/2
  Constant/1 -> Index Vector1/2
  Product2/1 -> Saturation/1(Mc_In)
  Demux/1 -> Mag_CmdCal/1(Cmd_Dir)
  Demux/2 -> Mux/1, Mag_CmdCal/2(Cmd_Cur)
  Cmd/1 -> Demux/1
  Saturation/1(Mc_Out) -> Mc_Mt/1, >=<0 to 012/1(In1), Abs3/1
  Constant2/1 -> Saturation/3(Mt_max_M)

== system GS_model/Subsystem2/Subsystem/Actuator/Magnetorquer/Mt_MathModel/MtA4 ==
  Tc_Mt : Inport
  Cmd : Inport  Port=2
  Mt_Num : Inport  Port=3
  >=<0 to 012 : Subsystem
  Abs3 : Abs
  Compare To Constant : simulink/Logic and Bit Operations/Compare To Constant  relop===  const=0  OutDataTypeStr=boolean
  Constant : Constant  Value=Mt_Cur2M
  Constant1 : Constant  Value=Mt_M2Cur
  Constant2 : Constant  Value=Mt_max_M
  Demux : Demux  Outputs=2
  Demux3 : Demux  Outputs=[1;2]
  Demux8 : Demux  Outputs=2
  If Action Subsystem3 : Subsystem  TreatAsAtomicUnit=on
  If Action Subsystem4 : Subsystem  TreatAsAtomicUnit=on
  If1 : If  IfExpression=u1 == 1
  Index Vector : MultiPortSwitch  Inputs=1
  Index Vector1 : MultiPortSwitch  Inputs=1
  Logical Operator : Logic  Operator=OR  AllPortsSameDT=off  OutDataTypeStr=boolean
  Mag_CmdCal : Subsystem
  Merge1 : Merge
  Mux : Mux  Inputs=2
  Mux1 : Mux  Inputs=2
  Product2 : Product
  Product3 : Product
  Relational Operator5 : RelationalOperator  Operator===  OutDataTypeStr=boolean  RndMeth=Simplest
  Saturation : MATLAB Function  TreatAsAtomicUnit=on
  Triggered Subsystem6 : Subsystem  TreatAsAtomicUnit=on
  Mc_Mt : Outport
  Tm_Mt : Outport  Port=2
  Cmd_Mt : Outport  Port=3
  wires:
  Constant2/1 -> Saturation/3(Mt_max_M)
  Saturation/1(Mc_Out) -> Abs3/1, >=<0 to 012/1(In1), Mc_Mt/1
  Cmd/1 -> Demux/1
  Demux/2 -> Mag_CmdCal/2(Cmd_Cur), Mux/1
  Demux/1 -> Mag_CmdCal/1(Cmd_Dir)
  Product2/1 -> Saturation/1(Mc_In)
  Constant/1 -> Index Vector1/2
  Merge1/1 -> Product2/2
  Index Vector1/1 -> Product2/1
  Compare To Constant/1 -> Logical Operator/1
  Logical Operator/1 -> Triggered Subsystem6/Enable
  Relational Operator5/1 -> Logical Operator/2
  Mt_Num/1 -> Relational Operator5/1, Saturation/2(Num), Index Vector1/1, Index Vector/1
  Constant1/1 -> Index Vector/2
  Demux8/2 -> If Action Subsystem4/1(In1)
  Mux1/1 -> Tm_Mt/1
  Mux/1 -> Cmd_Mt/1
  Mag_CmdCal/2(Cmd_Dirr) -> Mux/2
  If1/1 -> If Action Subsystem4/Action
  If1/2 -> If Action Subsystem3/Action
  Triggered Subsystem6/1(Out1) -> Demux8/1
  Demux3/2 -> Triggered Subsystem6/1(In1)
  Demux3/1 -> Relational Operator5/2, Compare To Constant/1
  If Action Subsystem3/1(Out1) -> Merge1/2
  Demux8/1 -> If1/1
  Tc_Mt/1 -> Demux3/1
  If Action Subsystem4/1(Out1) -> Merge1/1
  >=<0 to 012/1(Out1) -> Mux1/2
  Mag_CmdCal/1("Cmd_Curr ") -> If Action Subsystem3/1(In1)
  Abs3/1 -> Product3/2
  Index Vector/1 -> Product3/1
  Product3/1 -> Mux1/1

== system GS_model/Subsystem2/Subsystem/Actuator/Magnetorquer/Mt_MathModel/MtA5 ==
  Tc_Mt : Inport
  Cmd : Inport  Port=2
  Mt_Num : Inport  Port=3
  >=<0 to 012 : Subsystem
  Abs3 : Abs
  Compare To Constant : simulink/Logic and Bit Operations/Compare To Constant  relop===  const=0  OutDataTypeStr=boolean
  Constant : Constant  Value=Mt_Cur2M
  Constant1 : Constant  Value=Mt_M2Cur
  Constant2 : Constant  Value=Mt_max_M
  Demux : Demux  Outputs=2
  Demux3 : Demux  Outputs=[1;2]
  Demux8 : Demux  Outputs=2
  If Action Subsystem3 : Subsystem  TreatAsAtomicUnit=on
  If Action Subsystem4 : Subsystem  TreatAsAtomicUnit=on
  If1 : If  IfExpression=u1 == 1
  Index Vector : MultiPortSwitch  Inputs=1
  Index Vector1 : MultiPortSwitch  Inputs=1
  Logical Operator : Logic  Operator=OR  AllPortsSameDT=off  OutDataTypeStr=boolean
  Mag_CmdCal : Subsystem
  Merge1 : Merge
  Mux : Mux  Inputs=2
  Mux1 : Mux  Inputs=2
  Product2 : Product
  Product3 : Product
  Relational Operator5 : RelationalOperator  Operator===  OutDataTypeStr=boolean  RndMeth=Simplest
  Saturation : MATLAB Function  TreatAsAtomicUnit=on
  Triggered Subsystem6 : Subsystem  TreatAsAtomicUnit=on
  Mc_Mt : Outport
  Tm_Mt : Outport  Port=2
  Cmd_Mt : Outport  Port=3
  wires:
  Product3/1 -> Mux1/1
  Index Vector/1 -> Product3/1
  Abs3/1 -> Product3/2
  Mag_CmdCal/1("Cmd_Curr ") -> If Action Subsystem3/1(In1)
  >=<0 to 012/1(Out1) -> Mux1/2
  If Action Subsystem4/1(Out1) -> Merge1/1
  Tc_Mt/1 -> Demux3/1
  Demux8/1 -> If1/1
  If Action Subsystem3/1(Out1) -> Merge1/2
  Demux3/1 -> Compare To Constant/1, Relational Operator5/2
  Demux3/2 -> Triggered Subsystem6/1(In1)
  Triggered Subsystem6/1(Out1) -> Demux8/1
  If1/2 -> If Action Subsystem3/Action
  If1/1 -> If Action Subsystem4/Action
  Mag_CmdCal/2(Cmd_Dirr) -> Mux/2
  Mux/1 -> Cmd_Mt/1
  Mux1/1 -> Tm_Mt/1
  Demux8/2 -> If Action Subsystem4/1(In1)
  Constant1/1 -> Index Vector/2
  Mt_Num/1 -> Index Vector/1, Index Vector1/1, Saturation/2(Num), Relational Operator5/1
  Relational Operator5/1 -> Logical Operator/2
  Logical Operator/1 -> Triggered Subsystem6/Enable
  Compare To Constant/1 -> Logical Operator/1
  Index Vector1/1 -> Product2/1
  Merge1/1 -> Product2/2
  Constant/1 -> Index Vector1/2
  Product2/1 -> Saturation/1(Mc_In)
  Demux/1 -> Mag_CmdCal/1(Cmd_Dir)
  Demux/2 -> Mux/1, Mag_CmdCal/2(Cmd_Cur)
  Cmd/1 -> Demux/1
  Saturation/1(Mc_Out) -> Mc_Mt/1, >=<0 to 012/1(In1), Abs3/1
  Constant2/1 -> Saturation/3(Mt_max_M)

== system GS_model/Subsystem2/Subsystem/Actuator/Magnetorquer/Mt_MathModel/MtA6 ==
  Tc_Mt : Inport
  Cmd : Inport  Port=2
  Mt_Num : Inport  Port=3
  >=<0 to 012 : Subsystem
  Abs3 : Abs
  Compare To Constant : simulink/Logic and Bit Operations/Compare To Constant  relop===  const=0  OutDataTypeStr=boolean
  Constant : Constant  Value=Mt_Cur2M
  Constant1 : Constant  Value=Mt_M2Cur
  Constant2 : Constant  Value=Mt_max_M
  Demux : Demux  Outputs=2
  Demux3 : Demux  Outputs=[1;2]
  Demux8 : Demux  Outputs=2
  If Action Subsystem3 : Subsystem  TreatAsAtomicUnit=on
  If Action Subsystem4 : Subsystem  TreatAsAtomicUnit=on
  If1 : If  IfExpression=u1 == 1
  Index Vector : MultiPortSwitch  Inputs=1
  Index Vector1 : MultiPortSwitch  Inputs=1
  Logical Operator : Logic  Operator=OR  AllPortsSameDT=off  OutDataTypeStr=boolean
  Mag_CmdCal : Subsystem
  Merge1 : Merge
  Mux : Mux  Inputs=2
  Mux1 : Mux  Inputs=2
  Product2 : Product
  Product3 : Product
  Relational Operator5 : RelationalOperator  Operator===  OutDataTypeStr=boolean  RndMeth=Simplest
  Saturation : MATLAB Function  TreatAsAtomicUnit=on
  Triggered Subsystem6 : Subsystem  TreatAsAtomicUnit=on
  Mc_Mt : Outport
  Tm_Mt : Outport  Port=2
  Cmd_Mt : Outport  Port=3
  wires:
  Constant2/1 -> Saturation/3(Mt_max_M)
  Saturation/1(Mc_Out) -> Abs3/1, >=<0 to 012/1(In1), Mc_Mt/1
  Cmd/1 -> Demux/1
  Demux/2 -> Mag_CmdCal/2(Cmd_Cur), Mux/1
  Demux/1 -> Mag_CmdCal/1(Cmd_Dir)
  Product2/1 -> Saturation/1(Mc_In)
  Constant/1 -> Index Vector1/2
  Merge1/1 -> Product2/2
  Index Vector1/1 -> Product2/1
  Compare To Constant/1 -> Logical Operator/1
  Logical Operator/1 -> Triggered Subsystem6/Enable
  Relational Operator5/1 -> Logical Operator/2
  Mt_Num/1 -> Relational Operator5/1, Saturation/2(Num), Index Vector1/1, Index Vector/1
  Constant1/1 -> Index Vector/2
  Demux8/2 -> If Action Subsystem4/1(In1)
  Mux1/1 -> Tm_Mt/1
  Mux/1 -> Cmd_Mt/1
  Mag_CmdCal/2(Cmd_Dirr) -> Mux/2
  If1/1 -> If Action Subsystem4/Action
  If1/2 -> If Action Subsystem3/Action
  Triggered Subsystem6/1(Out1) -> Demux8/1
  Demux3/2 -> Triggered Subsystem6/1(In1)
  Demux3/1 -> Relational Operator5/2, Compare To Constant/1
  If Action Subsystem3/1(Out1) -> Merge1/2
  Demux8/1 -> If1/1
  Tc_Mt/1 -> Demux3/1
  If Action Subsystem4/1(Out1) -> Merge1/1
  >=<0 to 012/1(Out1) -> Mux1/2
  Mag_CmdCal/1("Cmd_Curr ") -> If Action Subsystem3/1(In1)
  Abs3/1 -> Product3/2
  Index Vector/1 -> Product3/1
  Product3/1 -> Mux1/1

== system GS_model/Subsystem2/Subsystem/Actuator/Motor/QV/Agl2Agl//w//a ==
  In1 : Inport
  Abs : Abs
  Delay : Delay  DelayLength=1  InitialCondition=0
  Discrete Derivative : simulink/Discrete/Discrete Derivative  gainval=1.0  ICPrevScaledInput=0.0  OutMin=[]  OutMax=[]  OutDataType=fixdt(1, 16)  OutScaling=2^-10  DoSatur=off
  Discrete Derivative3 : simulink/Discrete/Discrete Derivative  gainval=1.0  ICPrevScaledInput=0.0  OutMin=[]  OutMax=[]  OutDataType=fixdt(1, 16)  OutScaling=2^-10  DoSatur=off
  Mux1 : Mux  Inputs=3
  Switch : Switch  Criteria=u2 > Threshold  Threshold=10*pi/180
  Out1 : Outport
  wires:
  Mux1/1 -> Out1/1
  In1/1 -> Discrete Derivative/1, Mux1/1
  Discrete Derivative3/1 -> Mux1/3
  Delay/1 -> Switch/1
  Discrete Derivative/1 -> Switch/3, Abs/1
  Switch/1 -> Delay/1, Mux1/2, Discrete Derivative3/1
  Abs/1 -> Switch/2

== system GS_model/Subsystem2/Subsystem/Actuator/Motor/QV/Data_QV ==
  Constant1 : Constant  Value=TestMode
  Signal Specification : SignalSpecification  Dimensions=124
  Switch : Switch  Criteria=u2 > Threshold  Threshold=0.5
  out : Outport
  wires:
  Switch/1 -> out/1
  Constant1/1 -> Switch/2
  [Data_QV_Proj] -> Switch/1
  [Data_QV_Test] -> Signal Specification/1
  Signal Specification/1 -> Switch/3

== system GS_model/Subsystem2/Subsystem/Actuator/Motor/QV/Fre_QV ==
  Constant1 : Constant  Value=TestMode
  Delay : Delay  DelayLength=1
  Signal Specification : SignalSpecification  Dimensions=4
  Switch : Switch  Criteria=u2 > Threshold  Threshold=0.5
  out : Outport
  wires:
  Delay/1 -> out/1
  Switch/1 -> Delay/1
  Constant1/1 -> Switch/2
  [Fre_QV_Proj] -> Switch/1
  [Fre_QV_Test] -> Signal Specification/1
  Signal Specification/1 -> Switch/3

== system GS_model/Subsystem2/Subsystem/Actuator/Motor/QV/Limit±180deg ==
  In1 : Inport
  Constant10 : Constant  Value=[360;360;360;360]
  Constant11 : Constant  Value=[1;1;1;1]
  Constant12 : Constant  Value=[0;0;0;0]
  Gain : Gain  Gain=360
  Math Function : Math  Operator=mod  SaturateOnIntegerOverflow=on
  Subtract : Sum  Inputs=+-
  Switch : Switch  Criteria=u2 > Threshold  Threshold=180
  Out1 : Outport
  wires:
  Constant10/1 -> Math Function/2
  In1/1 -> Math Function/1
  Gain/1 -> Subtract/2
  Constant11/1 -> Switch/1
  Switch/1 -> Gain/1
  Subtract/1 -> Out1/1
  Math Function/1 -> Switch/2, Subtract/1
  Constant12/1 -> Switch/3

== system GS_model/Subsystem2/Subsystem/Actuator/Motor/QV/Subsystem ==
  note: St_Second
  note: St_MicroSecond
  UTC_1970 : Inport
  Add3 : Sum  Inputs=-+
  Constant : Constant  Value=QV_TimeStamp_leap
  Gain1 : Gain  Gain=1e06  SaturateOnIntegerOverflow=on  OutDataTypeStr=Inherit: Same as input  ParamDataTypeStr=Inherit: Same as input
  Mux : Mux  Inputs=2
  Rounding Function1 : Rounding
  Rounding Function2 : Rounding
  Sum : Sum  Inputs=|++
  St_Time : Outport
  wires:
  Rounding Function1/1 -> Add3/1, Mux/1
  Gain1/1 -> Rounding Function2/1
  Add3/1 -> Gain1/1
  Rounding Function2/1 -> Mux/2
  Mux/1 -> St_Time/1
  UTC_1970/1 -> Sum/1
  Constant/1 -> Sum/2
  Sum/1 -> Add3/2, Rounding Function1/1

== system GS_model/Subsystem2/Subsystem/Actuator/Motor/QV/Subsystem3 ==
  In1 : Inport
  Constant1 : Constant  Value=QV_Agl_HL1(1,:)'
  Constant2 : Constant  Value=QV_Agl_HL2(1,:)'
  Constant3 : Constant  Value=QV_Agl_HL2(2,:)'
  Constant4 : Constant  Value=QV_Agl_HL1(2,:)'
  Data Type Conversion : DataTypeConversion
  Data Type Conversion1 : DataTypeConversion
  Logical Operator : Logic  AllPortsSameDT=off  OutDataTypeStr=boolean
  Logical Operator1 : Logic  AllPortsSameDT=off  OutDataTypeStr=boolean
  Relational Operator : RelationalOperator  Operator=<=  OutDataTypeStr=boolean  RndMeth=Simplest
  Relational Operator1 : RelationalOperator  Operator=>  OutDataTypeStr=boolean  RndMeth=Simplest
  Relational Operator2 : RelationalOperator  Operator=<=  OutDataTypeStr=boolean  RndMeth=Simplest
  Relational Operator3 : RelationalOperator  Operator=>  OutDataTypeStr=boolean  RndMeth=Simplest
  DATA_Motor_HE1Sta : Outport
  DATA_Motor_HE2Sta : Outport  Port=2
  wires:
  Constant3/1 -> Relational Operator2/2
  Data Type Conversion1/1 -> DATA_Motor_HE2Sta/1
  In1/1 -> Relational Operator/1, Relational Operator1/1, Relational Operator2/1, Relational Operator3/1
  Data Type Conversion/1 -> DATA_Motor_HE1Sta/1
  Logical Operator1/1 -> Data Type Conversion1/1
  Relational Operator2/1 -> Logical Operator1/1
  Relational Operator3/1 -> Logical Operator1/2
  Constant2/1 -> Relational Operator3/2
  Relational Operator1/1 -> Logical Operator/2
  Relational Operator/1 -> Logical Operator/1
  Constant1/1 -> Relational Operator1/2
  Constant4/1 -> Relational Operator/2
  Logical Operator/1 -> Data Type Conversion/1

== system GS_model/Subsystem2/Subsystem/Actuator/Motor/SADA/Agl2Agl//w//a ==
  In1 : Inport
  Abs : Abs
  Delay : Delay  DelayLength=1  InitialCondition=0
  Discrete Derivative : simulink/Discrete/Discrete Derivative  gainval=1.0  ICPrevScaledInput=0.0  OutMin=[]  OutMax=[]  OutDataType=fixdt(1, 16)  OutScaling=2^-10  DoSatur=off
  Discrete Derivative3 : simulink/Discrete/Discrete Derivative  gainval=1.0  ICPrevScaledInput=0.0  OutMin=[]  OutMax=[]  OutDataType=fixdt(1, 16)  OutScaling=2^-10  DoSatur=off
  Mux1 : Mux  Inputs=3
  Switch : Switch  Criteria=u2 > Threshold  Threshold=10*pi/180
  Out1 : Outport
  wires:
  Abs/1 -> Switch/2
  Switch/1 -> Discrete Derivative3/1, Mux1/2, Delay/1
  Discrete Derivative/1 -> Abs/1, Switch/3
  Delay/1 -> Switch/1
  Discrete Derivative3/1 -> Mux1/3
  In1/1 -> Mux1/1, Discrete Derivative/1
  Mux1/1 -> Out1/1

== system GS_model/Subsystem2/Subsystem/Actuator/Motor/SADA/Data_SADA ==
  Constant1 : Constant  Value=TestMode
  Signal Specification : SignalSpecification  Dimensions=186
  Switch : Switch  Criteria=u2 > Threshold  Threshold=0.5
  out : Outport
  wires:
  [Data_SADA_Proj] -> Switch/1
  Constant1/1 -> Switch/2
  Switch/1 -> out/1
  [Data_SADA_Test] -> Signal Specification/1
  Signal Specification/1 -> Switch/3

== system GS_model/Subsystem2/Subsystem/Actuator/Motor/SADA/Fre_SADA ==
  Constant1 : Constant  Value=TestMode
  Delay : Delay  DelayLength=1
  Signal Specification : SignalSpecification  Dimensions=6
  Switch : Switch  Criteria=u2 > Threshold  Threshold=0.5
  out : Outport
  wires:
  [Fre_SADA_Proj] -> Switch/1
  Constant1/1 -> Switch/2
  Switch/1 -> Delay/1
  Delay/1 -> out/1
  [Fre_SADA_Test] -> Signal Specification/1
  Signal Specification/1 -> Switch/3

== system GS_model/Subsystem2/Subsystem/Actuator/Motor/SADA/Limit±180deg ==
  In1 : Inport
  Constant10 : Constant  Value=[360;360;360;360;360;360]
  Constant11 : Constant  Value=[1;1;1;1;1;1]
  Constant12 : Constant  Value=[0;0;0;0;0;0]
  Gain : Gain  Gain=360
  Math Function : Math  Operator=mod  SaturateOnIntegerOverflow=on
  Subtract : Sum  Inputs=+-
  Switch : Switch  Criteria=u2 > Threshold  Threshold=180
  Out1 : Outport
  wires:
  Constant12/1 -> Switch/3
  Math Function/1 -> Subtract/1, Switch/2
  Subtract/1 -> Out1/1
  Switch/1 -> Gain/1
  Constant11/1 -> Switch/1
  Gain/1 -> Subtract/2
  In1/1 -> Math Function/1
  Constant10/1 -> Math Function/2

== system GS_model/Subsystem2/Subsystem/Actuator/Motor/SADA/Subsystem ==
  note: St_Second
  note: St_MicroSecond
  UTC_1970 : Inport
  Add3 : Sum  Inputs=-+
  Constant : Constant  Value=SADA_TimeStamp_leap
  Gain1 : Gain  Gain=1e06  SaturateOnIntegerOverflow=on  OutDataTypeStr=Inherit: Same as input  ParamDataTypeStr=Inherit: Same as input
  Mux : Mux  Inputs=2
  Rounding Function1 : Rounding
  Rounding Function2 : Rounding
  Sum : Sum  Inputs=|++
  St_Time : Outport
  wires:
  Rounding Function1/1 -> Add3/1, Mux/1
  Gain1/1 -> Rounding Function2/1
  Add3/1 -> Gain1/1
  Rounding Function2/1 -> Mux/2
  Mux/1 -> St_Time/1
  UTC_1970/1 -> Sum/1
  Constant/1 -> Sum/2
  Sum/1 -> Add3/2, Rounding Function1/1

== system GS_model/Subsystem2/Subsystem/Actuator/Motor/SADA/Subsystem3 ==
  In1 : Inport
  Constant1 : Constant  Value=SADA_Agl_HL1(1,:)'
  Constant2 : Constant  Value=SADA_Agl_HL2(1,:)'
  Constant3 : Constant  Value=SADA_Agl_HL2(2,:)'
  Constant4 : Constant  Value=SADA_Agl_HL1(2,:)'
  Data Type Conversion : DataTypeConversion
  Data Type Conversion1 : DataTypeConversion
  Logical Operator : Logic  AllPortsSameDT=off  OutDataTypeStr=boolean
  Logical Operator1 : Logic  AllPortsSameDT=off  OutDataTypeStr=boolean
  Relational Operator : RelationalOperator  Operator=<=  OutDataTypeStr=boolean  RndMeth=Simplest
  Relational Operator1 : RelationalOperator  Operator=>  OutDataTypeStr=boolean  RndMeth=Simplest
  Relational Operator2 : RelationalOperator  Operator=<=  OutDataTypeStr=boolean  RndMeth=Simplest
  Relational Operator3 : RelationalOperator  Operator=>  OutDataTypeStr=boolean  RndMeth=Simplest
  DATA_Motor_HE1Sta : Outport
  DATA_Motor_HE2Sta : Outport  Port=2
  wires:
  Logical Operator/1 -> Data Type Conversion/1
  Constant4/1 -> Relational Operator/2
  Constant1/1 -> Relational Operator1/2
  Relational Operator/1 -> Logical Operator/1
  Relational Operator1/1 -> Logical Operator/2
  Constant2/1 -> Relational Operator3/2
  Relational Operator3/1 -> Logical Operator1/2
  Relational Operator2/1 -> Logical Operator1/1
  Logical Operator1/1 -> Data Type Conversion1/1
  Data Type Conversion/1 -> DATA_Motor_HE1Sta/1
  In1/1 -> Relational Operator3/1, Relational Operator2/1, Relational Operator1/1, Relational Operator/1
  Data Type Conversion1/1 -> DATA_Motor_HE2Sta/1
  Constant3/1 -> Relational Operator2/2

== system GS_model/Subsystem2/Subsystem/PhysicsModel/DynModel/Att：ECEF2VVLH/ECI TO ORBIT ==
  wbi(b) : Inport
  w00 : Inport  Port=2
  Abo : Inport  Port=3
  Constant : Constant  Value=0
  Gain : Gain  Gain=-1
  Matrix Multiply : Product  Multiplication=Matrix(*)
  Mux1 : Mux  Inputs=3
  Sum : Sum  Inputs=+|-
  wbo(b) : Outport
  wires:
  Matrix Multiply/1 -> Sum/2
  Sum/1 -> wbo(b)/1
  wbi(b)/1 -> Sum/1
  Abo/1 -> Matrix Multiply/1
  Gain/1 -> Mux1/2
  Constant/1 -> Mux1/1, Mux1/3
  w00/1 -> Gain/1
  Mux1/1 -> Matrix Multiply/2

== system GS_model/Subsystem2/Subsystem/PhysicsModel/DynModel/FlexDynModel/Agl_Qib ==
  Constant1 : Constant  Value=TestMode
  Delay : Delay  DelayLength=1
  Rotation Angles to Quaternions : sharedtransform/Rotation Angles to Quaternions  rotationOrder=ZYX  aMode=aMode
      settings: SourceProductBaseCode=AE,PW,MT,VE,VP
  Signal Specification : SignalSpecification  Dimensions=3
  Switch : Switch  Criteria=u2 > Threshold  Threshold=0.5
  out : Outport
  wires:
  Rotation Angles to Quaternions/1 -> out/1
  Constant1/1 -> Switch/2
  [Agl_Qib_Proj] -> Switch/1
  [Agl_Qib_Test] -> Signal Specification/1
  Switch/1 -> Delay/1
  Delay/1 -> Rotation Angles to Quaternions/1
  Signal Specification/1 -> Switch/3

== system GS_model/Subsystem2/Subsystem/PhysicsModel/DynModel/FlexDynModel/Cent ==
  Constant1 : Constant  Value=TestMode
  Delay : Delay  DelayLength=1
  Signal Specification : SignalSpecification  Dimensions=3
  Switch : Switch  Criteria=u2 > Threshold  Threshold=0.5
  out : Outport
  wires:
  Constant1/1 -> Switch/2
  [Cent_Proj] -> Switch/1
  Switch/1 -> Delay/1
  Delay/1 -> out/1
  [Cent_Test] -> Signal Specification/1
  Signal Specification/1 -> Switch/3

== system GS_model/Subsystem2/Subsystem/PhysicsModel/DynModel/FlexDynModel/I ==
  Constant1 : Constant  Value=TestMode
  Delay : Delay  DelayLength=1
  Reshape : Reshape  OutputDimensionality=Customize  OutputDimensions=[3,3]
  Signal Specification : SignalSpecification  Dimensions=9
  Switch : Switch  Criteria=u2 > Threshold  Threshold=0.5
  out : Outport
  wires:
  Reshape/1 -> out/1
  Constant1/1 -> Switch/2
  [I_Proj] -> Switch/1
  [I_Test] -> Signal Specification/1
  Switch/1 -> Delay/1
  Delay/1 -> Reshape/1
  Signal Specification/1 -> Switch/3

== system GS_model/Subsystem2/Subsystem/PhysicsModel/DynModel/FlexDynModel/R ==
  Constant1 : Constant  Value=TestMode
  Signal Specification : SignalSpecification  Dimensions=3
  Switch : Switch  Criteria=u2 > Threshold  Threshold=0.5
  out : Outport
  wires:
  Constant1/1 -> Switch/2
  [R_Proj] -> Switch/1
  Switch/1 -> out/1
  [R_Test] -> Signal Specification/1
  Signal Specification/1 -> Switch/3

== system GS_model/Subsystem2/Subsystem/PhysicsModel/DynModel/FlexDynModel/V ==
  Constant1 : Constant  Value=TestMode
  Signal Specification : SignalSpecification  Dimensions=3
  Switch : Switch  Criteria=u2 > Threshold  Threshold=0.5
  out : Outport
  wires:
  [V_Proj] -> Switch/1
  Constant1/1 -> Switch/2
  [V_Test] -> Signal Specification/1
  Switch/1 -> out/1
  Signal Specification/1 -> Switch/3

== system GS_model/Subsystem2/Subsystem/PhysicsModel/DynModel/FlexDynModel/dq ==
  Constant1 : Constant  Value=TestMode
  Signal Specification : SignalSpecification  Dimensions=10
  Switch : Switch  Criteria=u2 > Threshold  Threshold=0.5
  out : Outport
  wires:
  Constant1/1 -> Switch/2
  [dq_Proj] -> Switch/1
  Switch/1 -> out/1
  [dq_Test] -> Signal Specification/1
  Signal Specification/1 -> Switch/3

== system GS_model/Subsystem2/Subsystem/PhysicsModel/DynModel/FlexDynModel/q ==
  Constant1 : Constant  Value=TestMode
  Signal Specification : SignalSpecification  Dimensions=10
  Switch : Switch  Criteria=u2 > Threshold  Threshold=0.5
  out : Outport
  wires:
  Constant1/1 -> Switch/2
  [q_Proj] -> Switch/1
  Switch/1 -> out/1
  [q_Test] -> Signal Specification/1
  Signal Specification/1 -> Switch/3

== system GS_model/Subsystem2/Subsystem/PhysicsModel/DynModel/FlexDynModel/wbi ==
  Constant1 : Constant  Value=TestMode
  Delay : Delay  DelayLength=1
  Signal Specification : SignalSpecification  Dimensions=3
  Switch : Switch  Criteria=u2 > Threshold  Threshold=0.5
  out : Outport
  wires:
  [wbi_Proj] -> Switch/1
  Constant1/1 -> Switch/2
  Switch/1 -> Delay/1
  Delay/1 -> out/1
  [wbi_Test] -> Signal Specification/1
  Signal Specification/1 -> Switch/3
